simulink model "roll_attitude"  (R2017a)
settings: Solver=VariableStepAuto  StartTime=0.0  StopTime=50  RelTol=1e-3
undefined symbols (not defined in the file): a_phi1, a_phi2, delta_a_max, P
settings Model: Creator=pizzaslayer  LastModifiedBy=Parth

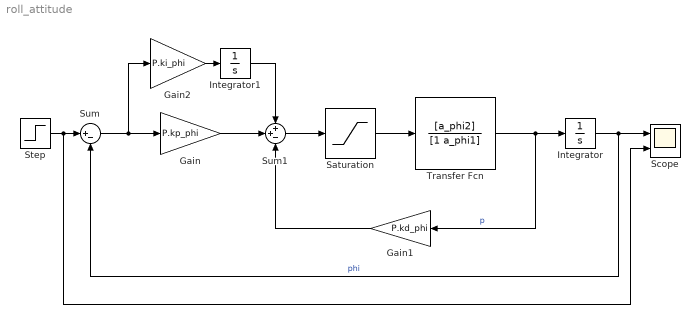
== system roll_attitude ==
  Gain : Gain  Gain=P.kp_phi
  Gain1 : Gain  Gain=P.kd_phi
  Gain2 : Gain  Gain=P.ki_phi
  Integrator : Integrator
  Integrator1 : Integrator
  Saturation : Saturate  UpperLimit=delta_a_max  LowerLimit=-delta_a_max
  Scope : Scope  NumInputPorts=2
  Step : Step  Time=0  SampleTime=0
  Sum : Sum  Inputs=|+-
  Sum1 : Sum  Inputs=++-
  Transfer Fcn : TransferFcn  Numerator=[a_phi2]  Denominator=[1 a_phi1]
  wires:
  Transfer Fcn/1 -> Gain1/1, Integrator/1  "p"
  Integrator/1 -> Sum/2, Scope/1  "phi"
  Step/1 -> Scope/2, Sum/1
  Sum/1 -> Gain2/1, Gain/1
  Gain/1 -> Sum1/2
  Gain1/1 -> Sum1/3
  Gain2/1 -> Integrator1/1
  Integrator1/1 -> Sum1/1
  Saturation/1 -> Transfer Fcn/1
  Sum1/1 -> Saturation/1
